simulink model "invpend"  (R2020b)
settings: Solver=FixedStepDiscrete  StartTime=0.0  StopTime=20  FixedStep=0.0001  RelTol=1e-3
values from neighbouring files (symbols this model uses):
  invpend_cart_mass = 5    [init_invpend.m]
  invpend_friction_coeff = 5    [init_invpend.m]
  invpend_pendulum_init_angle = invpend_pendulum_init_angle_in_deg * pi / 180    (= 0.13962634016)    [init_invpend.m]
  invpend_pendulum_length = 1.5    [init_invpend.m]
  invpend_pendulum_mass = 3    [init_invpend.m]
  invpend_pid_derivative_gain = 20    [init_invpend.m]
  invpend_pid_integral_gain = 60    [init_invpend.m]
  invpend_pid_proportional_gain = 100    [init_invpend.m]
  invpend_use_controller = true    [init_invpend.m]
  invpend_use_resistance = true    [init_invpend.m]    (also in result_visualizer.m)
undefined symbols (not defined in the file or in its folder): DiscIntNeverNeededParam
libraries: pid_lib x1
settings Model: Creator=kacskovt  LastModifiedBy=kacskovt

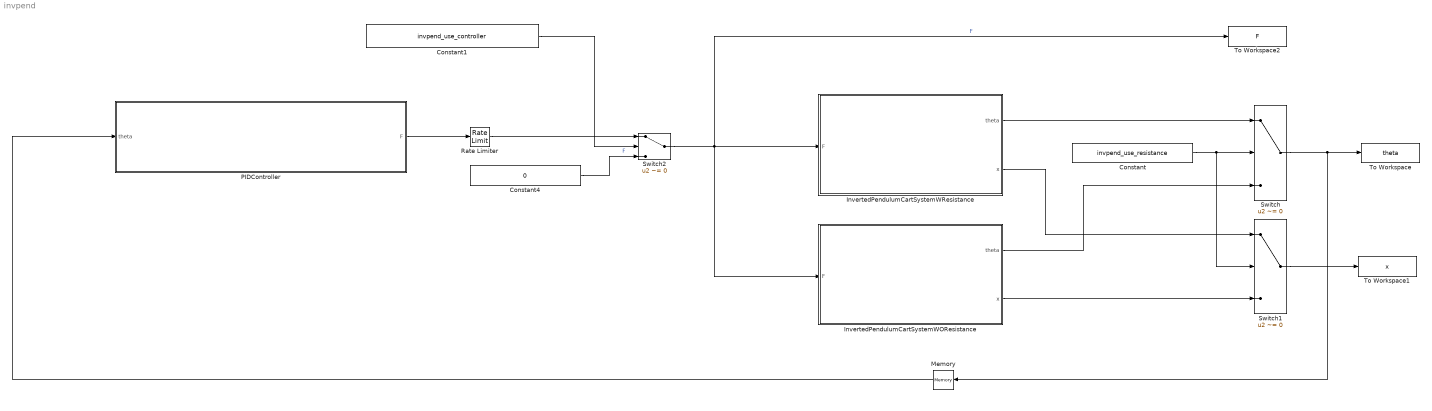
== system invpend ==
  Constant : Constant  Value=invpend_use_resistance
  Constant1 : Constant  Value=invpend_use_controller
  Constant4 : Constant  Value=0
  InvertedPendulumCartSystemWOResistance : Subsystem
  InvertedPendulumCartSystemWResistance : Subsystem
  Memory : Memory
  PIDController : Subsystem
  Rate Limiter : RateLimiter  RisingSlewLimit=100  FallingSlewLimit=-100  SampleTimeMode=inherited
  Switch : Switch  Criteria=u2 ~= 0
  Switch1 : Switch  Criteria=u2 ~= 0
  Switch2 : Switch  Criteria=u2 ~= 0
  To Workspace : ToWorkspace  VariableName=theta  SaveFormat=Timeseries  SampleTime=-1
  To Workspace1 : ToWorkspace  VariableName=x  SaveFormat=Timeseries  SampleTime=-1
  To Workspace2 : ToWorkspace  VariableName=F  SaveFormat=Timeseries  SampleTime=-1
  wires:
  InvertedPendulumCartSystemWResistance/1(theta) -> Switch/1
  InvertedPendulumCartSystemWResistance/2(x) -> Switch1/1
  InvertedPendulumCartSystemWOResistance/1(theta) -> Switch/3
  InvertedPendulumCartSystemWOResistance/2(x) -> Switch1/3
  Switch1/1 -> To Workspace1/1
  Switch/1 -> Memory/1, To Workspace/1
  Constant/1 -> Switch1/2, Switch/2
  Constant4/1 -> Switch2/3  "F"
  Switch2/1 -> InvertedPendulumCartSystemWOResistance/1(F), To Workspace2/1, InvertedPendulumCartSystemWResistance/1(F)  "F"
  Memory/1 -> PIDController/1(theta)
  PIDController/1(F) -> Rate Limiter/1
  Constant1/1 -> Switch2/2
  Rate Limiter/1 -> Switch2/1

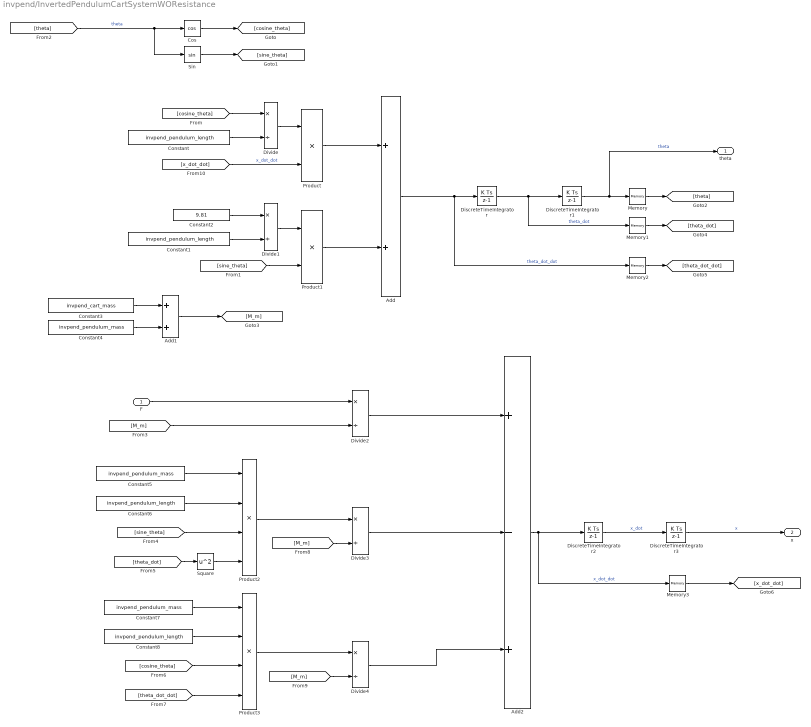
== system invpend/InvertedPendulumCartSystemWOResistance ==
  F : Inport
  Add : Sum
  Add1 : Sum
  Add2 : Sum  Inputs=+-+
  Constant{,1,6,8} (4 alike) : Constant  Value=invpend_pendulum_length
  Constant2 : Constant  Value=9.81
  Constant3 : Constant  Value=invpend_cart_mass
  Constant4 : Constant  Value=invpend_pendulum_mass
  Constant5 : Constant  Value=invpend_pendulum_mass
  Constant7 : Constant  Value=invpend_pendulum_mass
  Cos : Trigonometry  Operator=cos
  DiscreteTimeIntegrator : DiscreteIntegrator  SampleTime=-1  ICPrevOutput=DiscIntNeverNeededParam  ICPrevScaledInput=DiscIntNeverNeededParam
  DiscreteTimeIntegrator1 : DiscreteIntegrator  InitialCondition=invpend_pendulum_init_angle  SampleTime=-1  ICPrevOutput=DiscIntNeverNeededParam  ICPrevScaledInput=DiscIntNeverNeededParam
  DiscreteTimeIntegrator2 : DiscreteIntegrator  SampleTime=-1  ICPrevOutput=DiscIntNeverNeededParam  ICPrevScaledInput=DiscIntNeverNeededParam
  DiscreteTimeIntegrator3 : DiscreteIntegrator  SampleTime=-1  ICPrevOutput=DiscIntNeverNeededParam  ICPrevScaledInput=DiscIntNeverNeededParam
  Divide{,1..4} (5 alike) : Product  Inputs=*/
  Memory{,1..3} (4 alike) : Memory
  Product : Product
  Product1 : Product
  Product2 : Product  Inputs=4
  Product3 : Product  Inputs=4
  Sin : Trigonometry
  Square : Math  Operator=square  SaturateOnIntegerOverflow=on
  theta : Outport
  x : Outport  Port=2
  wires:
  Cos/1 -> [cosine_theta]
  Sin/1 -> [sine_theta]
  [theta] -> Sin/1, Cos/1  "theta"
  [cosine_theta] -> Divide/1
  Constant/1 -> Divide/2
  Divide/1 -> Product/1
  [x_dot_dot] -> Product/2  "x_dot_dot"
  Constant1/1 -> Divide1/2
  Constant2/1 -> Divide1/1
  Divide1/1 -> Product1/1
  [sine_theta] -> Product1/2
  Product/1 -> Add/1
  Product1/1 -> Add/2
  Add/1 -> Memory2/1, DiscreteTimeIntegrator/1  "theta_dot_dot"
  DiscreteTimeIntegrator/1 -> Memory1/1, DiscreteTimeIntegrator1/1  "theta_dot"
  DiscreteTimeIntegrator1/1 -> theta/1, Memory/1  "theta"
  F/1 -> Divide2/1
  Constant3/1 -> Add1/1
  Constant4/1 -> Add1/2
  Add1/1 -> [M_m]
  [M_m] -> Divide2/2
  Constant5/1 -> Product2/1
  Constant6/1 -> Product2/2
  [sine_theta] -> Product2/3
  Memory/1 -> [theta]
  [theta_dot] -> Square/1
  Square/1 -> Product2/4
  Constant7/1 -> Product3/1
  Constant8/1 -> Product3/2
  [cosine_theta] -> Product3/3
  Memory1/1 -> [theta_dot]
  Memory2/1 -> [theta_dot_dot]
  [theta_dot_dot] -> Product3/4
  Product2/1 -> Divide3/1
  [M_m] -> Divide3/2
  Product3/1 -> Divide4/1
  [M_m] -> Divide4/2
  Divide2/1 -> Add2/1
  Divide3/1 -> Add2/2
  Divide4/1 -> Add2/3
  Add2/1 -> Memory3/1, DiscreteTimeIntegrator2/1  "x_dot_dot"
  DiscreteTimeIntegrator2/1 -> DiscreteTimeIntegrator3/1  "x_dot"
  DiscreteTimeIntegrator3/1 -> x/1  "x"
  Memory3/1 -> [x_dot_dot]

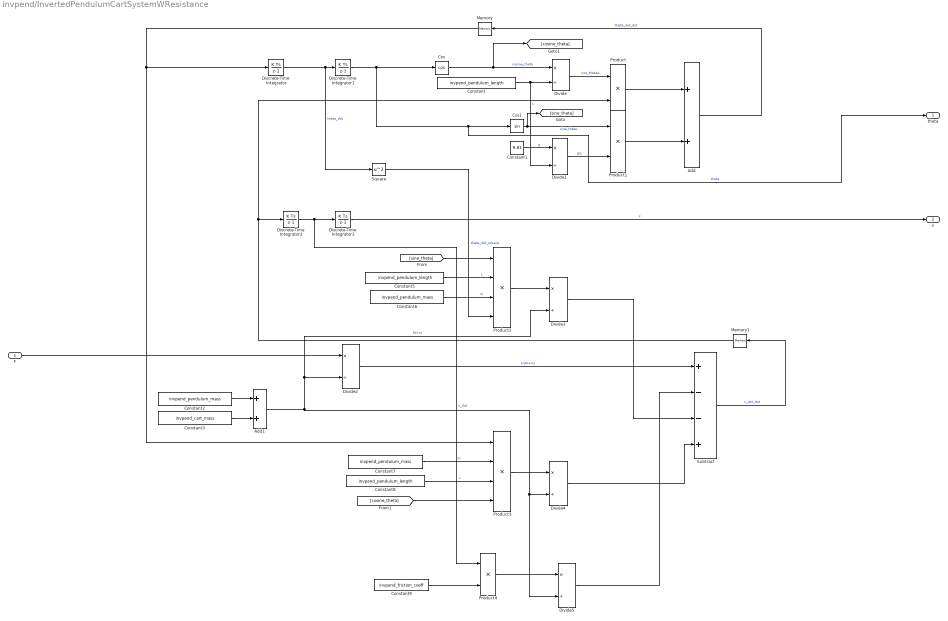
== system invpend/InvertedPendulumCartSystemWResistance ==
  F : Inport
  Add : Sum
  Add1 : Sum
  Constant : Constant  Value=invpend_pendulum_length
  Constant1 : Constant  Value=9.81
  Constant2 : Constant  Value=invpend_pendulum_mass
  Constant3 : Constant  Value=invpend_cart_mass
  Constant5 : Constant  Value=invpend_pendulum_length
  Constant6 : Constant  Value=invpend_pendulum_mass
  Constant7 : Constant  Value=invpend_pendulum_mass
  Constant8 : Constant  Value=invpend_pendulum_length
  Constant9 : Constant  Value=invpend_friction_coeff
  Cos : Trigonometry  Operator=cos
  Cos1 : Trigonometry
  Discrete-Time Integrator : DiscreteIntegrator  SampleTime=-1  ICPrevOutput=DiscIntNeverNeededParam  ICPrevScaledInput=DiscIntNeverNeededParam
  Discrete-Time Integrator1 : DiscreteIntegrator  InitialCondition=invpend_pendulum_init_angle  SampleTime=-1  ICPrevOutput=DiscIntNeverNeededParam  ICPrevScaledInput=DiscIntNeverNeededParam
  Discrete-Time Integrator2 : DiscreteIntegrator  SampleTime=-1  ICPrevOutput=DiscIntNeverNeededParam  ICPrevScaledInput=DiscIntNeverNeededParam
  Discrete-Time Integrator3 : DiscreteIntegrator  SampleTime=-1  ICPrevOutput=DiscIntNeverNeededParam  ICPrevScaledInput=DiscIntNeverNeededParam
  Divide{,1..5} (6 alike) : Product  Inputs=*/
  Memory : Memory
  Memory1 : Memory
  Product : Product
  Product1 : Product
  Product2 : Product  Inputs=4
  Product3 : Product  Inputs=4
  Product4 : Product
  Square : Math  Operator=square  SaturateOnIntegerOverflow=on
  Subtract : Sum  Inputs=+--+
  theta : Outport
  x : Outport  Port=2
  wires:
  Discrete-Time Integrator2/1 -> Discrete-Time Integrator3/1, Product4/1  "x_dot"
  Cos1/1 -> Product1/1, [sine_theta]  "sine_theta"
  [sine_theta] -> Product2/1
  Constant1/1 -> Divide1/1  "g"
  Product3/1 -> Divide4/1
  Memory/1 -> Discrete-Time Integrator/1, Product3/1
  F/1 -> Divide2/1
  Divide3/1 -> Subtract/3
  Discrete-Time Integrator/1 -> Discrete-Time Integrator1/1, Square/1  "theta_dot"
  Square/1 -> Product2/4  "theta_dot_square"
  Divide2/1 -> Subtract/1  "F/(M+m)"
  Product1/1 -> Add/2
  Memory1/1 -> Discrete-Time Integrator2/1, Product/2
  Constant/1 -> Divide1/2, Divide/2  "L"
  Constant5/1 -> Product2/2  "L"
  Cos/1 -> [cosine_theta], Divide/1  "cosine_theta"
  Divide1/1 -> Product1/2  "g/L"
  Add1/1 -> Divide5/2, Divide4/2, Divide3/2, Divide2/2  "M+m"
  Discrete-Time Integrator1/1 -> Cos/1, theta/1, Cos1/1  "theta"
  Subtract/1 -> Memory1/1  "x_dot_dot"
  Product4/1 -> Divide5/1
  Constant7/1 -> Product3/2  "m"
  Divide/1 -> Product/1  "cos_theta/L"
  Constant9/1 -> Product4/2
  Constant2/1 -> Add1/1
  Product/1 -> Add/1
  Constant3/1 -> Add1/2
  Constant8/1 -> Product3/3  "L"
  Add/1 -> Memory/1  "theta_dot_dot"
  [cosine_theta] -> Product3/4
  Product2/1 -> Divide3/1
  Constant6/1 -> Product2/3  "m"
  Discrete-Time Integrator3/1 -> x/1  "x"
  Divide4/1 -> Subtract/4
  Divide5/1 -> Subtract/2

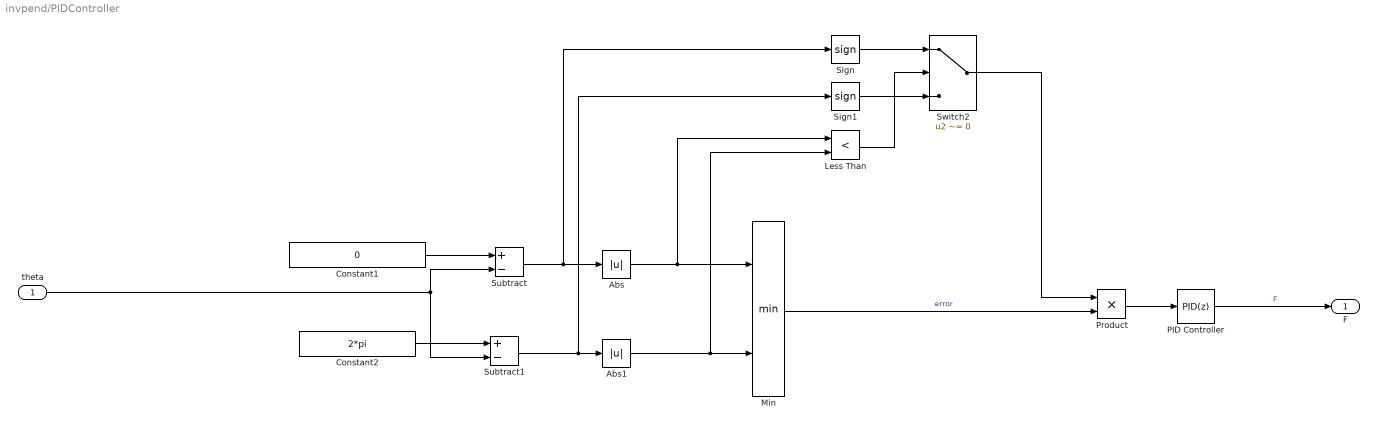
== system invpend/PIDController ==
  theta : Inport
  Abs : Abs
  Abs1 : Abs
  Constant1 : Constant  Value=0
  Constant2 : Constant  Value=2*pi
  Less Than : RelationalOperator  Operator=<  OutDataTypeStr=boolean  RndMeth=Simplest
  Min : MinMax  Inputs=2
  PID Controller : pid_lib/PID Controller  Controller=PID  Form=Parallel  TimeDomain=Discrete-time  UseExternalTs=off  SampleTime=-1  IntegratorMethod=Forward Euler  FilterMethod=Forward Euler  ControllerParametersSource=internal  P=invpend_pid_proportional_gain  I=invpend_pid_integral_gain  D=invpend_pid_derivative_gain  UseFilter=on  N=100  TunerSelectOption=Transfer Function Based (PID Tuner App)  InitialConditionSource=internal  InitialConditionForIntegrator=0  InitialConditionForFilter=0  DifferentiatorICPrevScaledInput=0  ExternalReset=none  TrackingMode=off  Kt=1  LimitOutput=off  SatLimitsSource=internal  UpperSaturationLimit=inf  LowerSaturationLimit=-inf  LinearizeAsGain=on  AntiWindupMode=none  Kb=1  POutMin=[]  POutMax=[]  IOutMin=[]  IOutMax=[]  DOutMin=[]  DOutMax=[]  NOutMin=[]  NOutMax=[]  SumOutMin=[]  SumOutMax=[]  SaturationOutMin=[]  SaturationOutMax=[]  PParamMin=[]  PParamMax=[]  IParamMin=[]  IParamMax=[]  DParamMin=[]  DParamMax=[]  NParamMin=[]  NParamMax=[]  KbParamMin=[]  KbParamMax=[]  KtParamMin=[]  KtParamMax=[]  KbOutMin=[]  KbOutMax=[]  KtOutMin=[]  KtOutMax=[]  IntegratorOutMin=[]  IntegratorOutMax=[]  FilterOutMin=[]  FilterOutMax=[]  SumI1OutMin=[]  SumI1OutMax=[]  SumI2OutMin=[]  SumI2OutMax=[]  SumI3OutMin=[]  SumI3OutMax=[]  SumI4OutMin=[]  SumI4OutMax=[]  SumDOutMin=[]  SumDOutMax=[]  DifferentiatorOutMin=[]  DifferentiatorOutMax=[]  FilterDiffOutCoefMin=[]  FilterDiffOutCoefMax=[]  ReciprocalOutMin=[]  ReciprocalOutMax=[]  SumDenOutMin=[]  SumDenOutMax=[]  SumNumOutMin=[]  SumNumOutMax=[]  DivideOutMin=[]  DivideOutMax=[]  UdiffTsProdOutMin=[]  UdiffTsProdOutMax=[]  NTsProdOutMin=[]  NTsProdOutMax=[]  UintegralTsProdOutMin=[]  UintegralTsProdOutMax=[]  UngainTsProdOutMin=[]  UngainTsProdOutMax=[]  IntegratorContinuousStateAttributes=''  IntegratorStateMustResolveToSignalObject=off  IntegratorRTWStateStorageClass=Auto  FilterContinuousStateAttributes=''  FilterStateMustResolveToSignalObject=off  FilterRTWStateStorageClass=Auto  ParallelPVariant=InternalParameters  IdealPVariant=Disabled  IVariant=InternalParameters  DVariant=InternalParameters  IntegratorVariant=Discrete  SatVariant=Disabled  AWVariant=Passthrough  PCopyVariant=Disabled  TRVariant=Disabled  FdbkBlocksVariant=Forward  IdealPFdbkVariant=Disabled  SatFdbkVariant=Disabled  DerivativeFilterVariant=ForwardEulerFilter  NVariant=InternalParameters  NCopyVariant=Disabled  FilterICVariant=InternalICsFilter  IntegratorICVariant=InternalICs  ExternalResetVariant=Disabled  TRSumVariant=Passthrough  SumFdbkVariant=Disabled  SumVariant=Sum_PID  TsampFilterVariant=InternalTs  TsampNgainVariant=Passthrough  TsampIntegralVariant=Passthrough  ExternalSaturationOutDataTypeStr=Inherit: Same as second input
  Product : Product
  Sign : Signum
  Sign1 : Signum
  Subtract : Sum  Inputs=+-
  Subtract1 : Sum  Inputs=+-
  Switch2 : Switch  Criteria=u2 ~= 0
  F : Outport
  wires:
  Abs/1 -> Min/1, Less Than/1
  Subtract1/1 -> Sign1/1, Abs1/1
  Switch2/1 -> Product/1
  Product/1 -> PID Controller/1
  Abs1/1 -> Less Than/2, Min/2
  PID Controller/1 -> F/1  "F"
  Sign1/1 -> Switch2/3
  Subtract/1 -> Sign/1, Abs/1
  theta/1 -> Subtract1/2, Subtract/2
  Min/1 -> Product/2  "error"
  Less Than/1 -> Switch2/2
  Sign/1 -> Switch2/1
  Constant1/1 -> Subtract/1
  Constant2/1 -> Subtract1/1
